simulink model "motordc"  (R2022a)
settings: Solver=VariableStepAuto  StartTime=0.0  StopTime=10.0  RelTol=1e-3
settings Model: Creator=User  LastModifiedBy=User

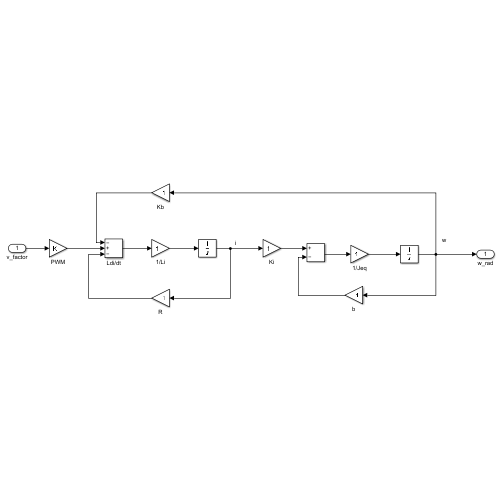
[thumbnail: Simulink's stored preview of the top-level diagram]
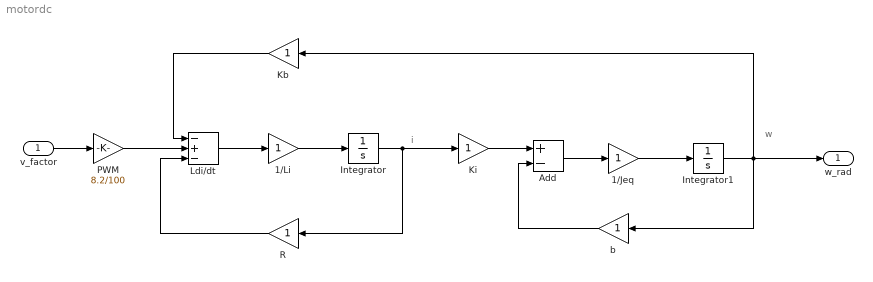
== system motordc ==
  note: w
  note: i
  v_factor : Inport
  1/Jeq : Gain
  1/Li : Gain
  Add : Sum  Inputs=+-
  Integrator : Integrator
  Integrator1 : Integrator
  Kb : Gain
  Ki : Gain
  Ldi/dt : Sum  Inputs=-+-
  PWM : Gain  Gain=8.2/100
  R : Gain
  b : Gain
  w_rad : Outport
  wires:
  v_factor/1 -> PWM/1
  PWM/1 -> Ldi/dt/2
  Ldi/dt/1 -> 1/Li/1
  1/Li/1 -> Integrator/1
  Integrator/1 -> Ki/1, R/1
  R/1 -> Ldi/dt/3
  Kb/1 -> Ldi/dt/1
  Ki/1 -> Add/1
  b/1 -> Add/2
  Add/1 -> 1/Jeq/1
  1/Jeq/1 -> Integrator1/1
  Integrator1/1 -> w_rad/1, Kb/1, b/1
